simulink model "trajectory2"  (R2024b)
settings: Solver=FixedStepAuto  StartTime=0.0  StopTime=inf  RelTol=1e-3
undefined symbols (not defined in the file): angular, linear
libraries: ros2lib x3
settings Model: Creator=advance_control_lab  LastModifiedBy=advance_control_lab
settings OptimizationCC: DefaultParameterBehavior=Inlined  EnhancedBackFolding=on  PassReuseOutputArgsAs=Individual arguments  ZeroExternalMemoryAtStartup=off  ZeroInternalMemoryAtStartup=off  MaxStackSize=64  OptimizeBlockOrder=speed  DifferentSizesBufferReuse=on  OptimizationCustomize=off  EfficientTunableParamExpr=on
settings DebuggingCC: ParameterTunabilityLossMsg=error
settings HardwareCC: ProdBitPerLong=64  ProdHWDeviceType=Intel->x86-64 (Linux 64)
settings SFSimCC: MATLABDynamicMemAlloc=off
settings RTWCC: Description=Embedded Coder  SystemTargetFile=ert.tlc  HardwareBoard=Robot Operating System 2 (ROS 2)  TLCOptions="-aInlineSetEventsForThisBaseRateFcn=TLC_FALSE -aSuppressMultiTaskScheduler=TLC_FALSE  -aRateBasedStepFcn=0"  GenCodeOnly=on  TemplateMakefile=ert_default_tmf  Toolchain=Colcon Tools  TargetLang=C++
settings CodeAppCC: ForceParamTrailComments=on  IgnoreCustomStorageClasses=off  OperatorAnnotations=on  SimulinkDataObjDesc=on  SFDataObjDesc=on  InsertBlockDesc=on
settings ERTTargetCC: CodeInterfacePackaging=C++ class  SupportVariableSizeSignals=on  RootIOFormat=Structure reference

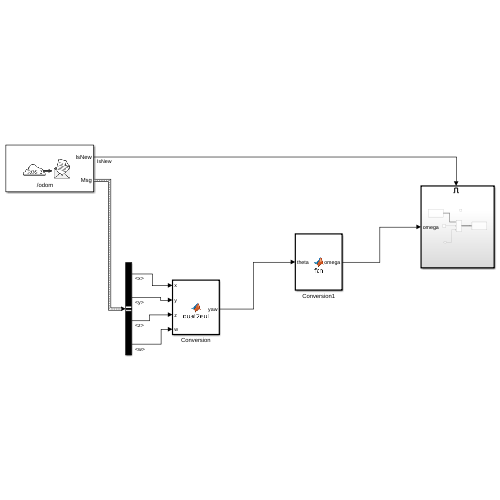
[thumbnail: Simulink's stored preview of the top-level diagram]
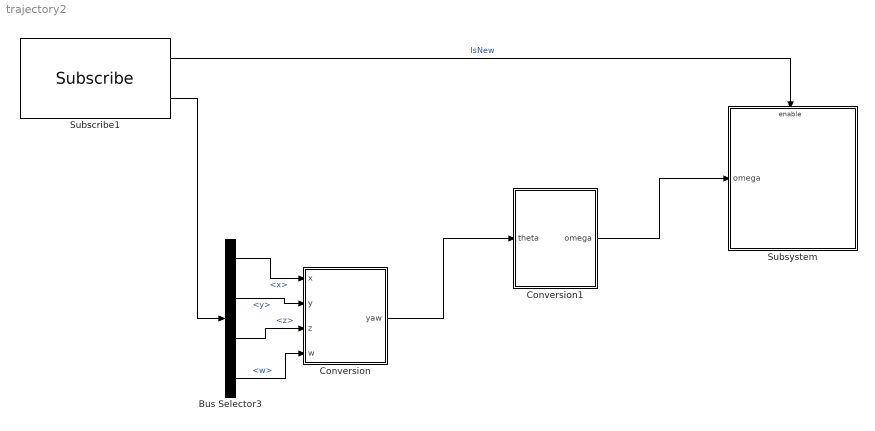
== system trajectory2 ==
  Bus Selector3 : BusSelector  OutputSignals=pose.pose.orientation.x,pose.pose.orientation.y,pose.pose.orientation.z,pose.pose.orientation.w
  Conversion : MATLAB Function  TreatAsAtomicUnit=on
  Conversion1 : MATLAB Function  TreatAsAtomicUnit=on
  Subscribe1 : ros2lib/Subscribe  topicSource=Specify your own  topic=/odom  messageType=nav_msgs/Odometry  sampleTime=-1  QOSHistory=Keep last  QOSDepth=1  QOSReliability=Reliable  QOSDurability=Volatile  QOSDeadline=Inf  QOSLifespan=Inf  QOSLiveliness=Automatic  QOSLeaseDuration=Inf  QOSAvoidROSNamespaceConventions=off
  Subsystem : Subsystem
  wires:
  Conversion/1(yaw) -> Conversion1/1(theta)
  Bus Selector3/1 -> Conversion/1(x)  "<x>"
  Conversion1/1(omega) -> Subsystem/1(omega)
  Subscribe1/1 -> Subsystem/Enable  "IsNew"
  Bus Selector3/4 -> Conversion/4(w)  "<w>"
  Bus Selector3/3 -> Conversion/3(z)  "<z>"
  Subscribe1/2 -> Bus Selector3/1
  Bus Selector3/2 -> Conversion/2(y)  "<y>"

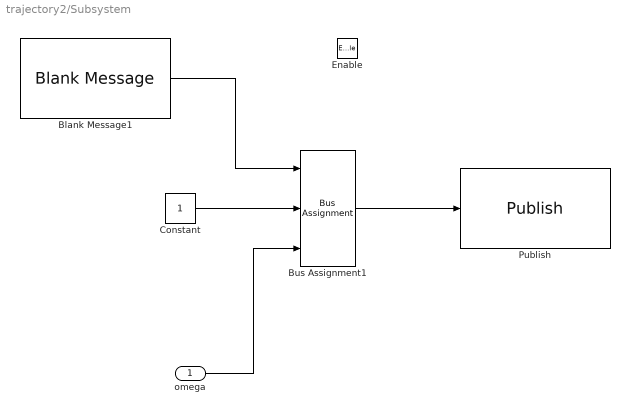
== system trajectory2/Subsystem ==
  omega : Inport
  Enable : EnablePort
  Blank Message1 : ros2lib/Blank Message  messageClass=Message  entityType=geometry_msgs/Twist  messageType=geometry_msgs/Twist  SampleTime=inf
  Bus Assignment1 : BusAssignment  DialogController=Simulink.DDGSource_BusAssignment  AssignedSignals=linear.x,angular.z
  Constant : Constant
  Publish : ros2lib/Publish  topicSource=Specify your own  topic=/cmd_vel  messageType=geometry_msgs/Twist  QOSHistory=Keep last  QOSDepth=1  QOSReliability=Reliable  QOSDurability=Volatile  QOSDeadline=Inf  QOSLifespan=Inf  QOSLiveliness=Automatic  QOSLeaseDuration=Inf  QOSAvoidROSNamespaceConventions=off
  wires:
  Bus Assignment1/1 -> Publish/1
  Blank Message1/1 -> Bus Assignment1/1
  Constant/1 -> Bus Assignment1/2
  omega/1 -> Bus Assignment1/3

== matlab function trajectory2/Conversion ==
  data: yaw output; x input; y input; z input; w input
function yaw  = quat2eul(x,y,z,w)
%#codegen

% Convert the quaternion to a yaw angle (zyx euler angle)
eul = quat2eul([w,x,y,z]);
yaw = eul(1);

end

== matlab function trajectory2/Conversion1 ==
  data: omega output; theta input
function omega = fcn(theta)
    % Inputs: theta (current value)
    % Outputs: omega (control signal)
    
    persistent direction;
    
    % Initialize the persistent variable on the first call
    if isempty(direction)
        direction = 1; % Initial direction: increasing
    end

    
    % Instead, check if theta is within the range and maintain omega.
    if (theta > -3 && theta < 0) || (theta > 0 && theta < 3)
        if direction == 1 && (theta > 0 && theta < 3)
            omega = 0.5;
            direction = 1;
        elseif direction == -1 && (theta > 0 && theta < 3)
            omega = -0.5;
            direction = -1;
        elseif direction == 1 && (theta > -3 && theta < 0)
            omega = 0.5;
            direction = 1;
        else 
            omega = -0.5;
            direction = -1;
            endsz
        return; % Exit the function to avoid further checks
    end

    % Control logic for boundary conditions
    if theta >= 3 
        omega = -0.5;   % Start decreasing theta
        direction = -1; % Change direction to decreasing
    elseif theta <= -3 
        omega = 0.5;    % Start increasing theta
        direction = 1;  % Change direction to increasing
    else
        
            omega = 0.5;
        
    end
end
